simulink model "PMSM_z_domain_HDL"  (R2019b)
settings: Solver=ode1  StartTime=0.0  StopTime=2  FixedStep=1e-5  RelTol=1e-3
InitFcn:
  | %T=0.0000071
  | T = (1e-5)/2
  | 
  | flux=0.2068
values from neighbouring files (symbols this model uses):
  B = 0.0136    [Pmsm.m]
  J = 0.0027    [Pmsm.m]
  Kiq = double(Kiq)    [Pmsm.m]
  Kiw = double(Kiw)    [Pmsm.m]
  Kpq = double(Kpq)    [Pmsm.m]
  Kpw = double(Kpw)    [Pmsm.m]
  Lambda_m = 0.2026    [Pmsm.m]
  Ld = 19.75e-3    (= 0.01975)    [Pmsm.m]
  Lq = 22.5e-3    (= 0.0225)    [Pmsm.m]
  Ls = (Ld+Lq)/2    (= 0.021125)    [Pmsm.m]
  P = 8    [Pmsm.m]
  Rs = 1.477    [Pmsm.m]
  Vdc = 220    [Pmsm.m]
libraries: powerlib_meascontrol x3
settings Model: Creator=samfi  LastModifiedBy=samfi

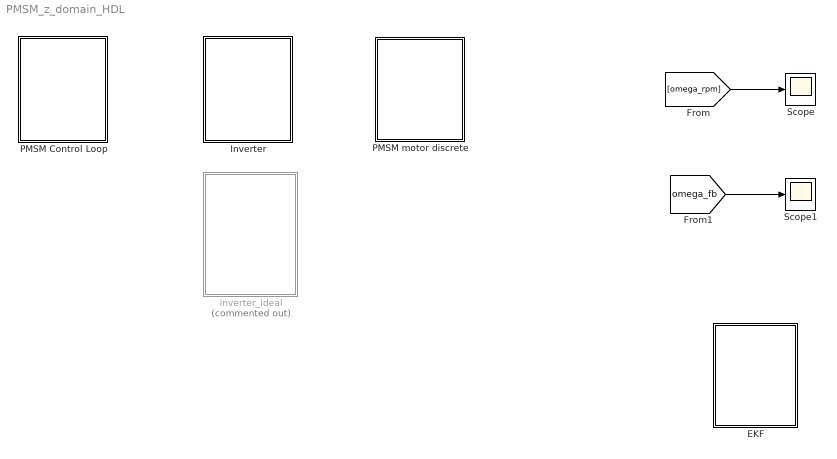
== system PMSM_z_domain_HDL ==
  EKF : Subsystem
  Inverter : Subsystem
  PMSM Control Loop : Subsystem
  PMSM motor discrete : Subsystem
  Scope : Scope
  Scope1 : Scope
  inverter_ideal : Subsystem  Commented=on
  wires:
  [omega_rpm] -> Scope/1
  [omega_fb] -> Scope1/1

== system PMSM_z_domain_HDL/EKF ==
  EKF good : Subsystem  Commented=on
  EKF good1 : Subsystem

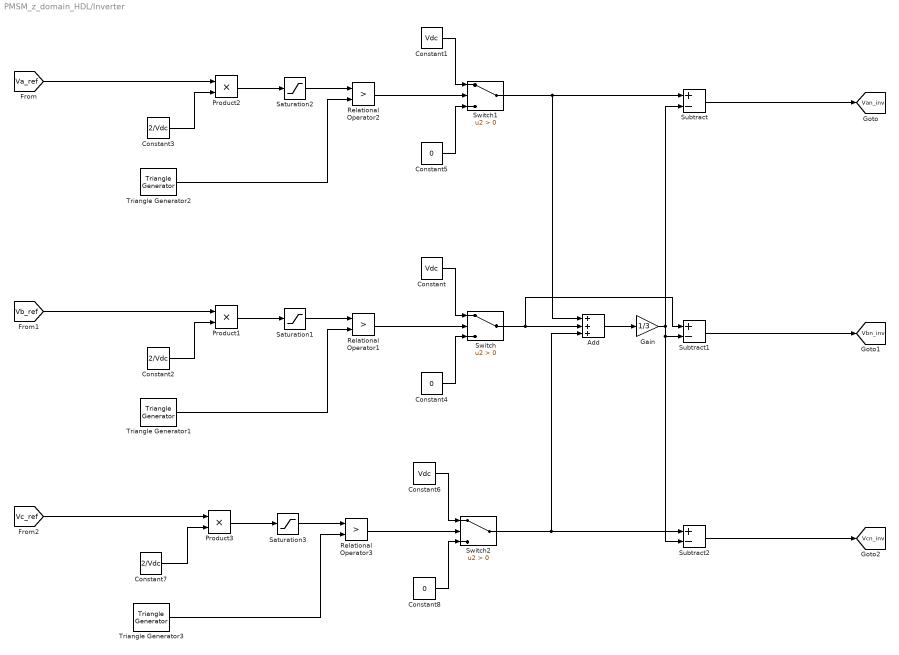
== system PMSM_z_domain_HDL/Inverter ==
  Add : Sum  Inputs=+++
  Constant : Constant  Value=Vdc
  Constant1 : Constant  Value=Vdc
  Constant2 : Constant  Value=2/Vdc
  Constant3 : Constant  Value=2/Vdc
  Constant4 : Constant  Value=0
  Constant5 : Constant  Value=0
  Constant6 : Constant  Value=Vdc
  Constant7 : Constant  Value=2/Vdc
  Constant8 : Constant  Value=0
  Gain : Gain  Gain=1/3
  Product1 : Product
  Product2 : Product
  Product3 : Product
  Relational Operator1 : RelationalOperator  Operator=>  OutDataTypeStr=boolean  RndMeth=Simplest
  Relational Operator2 : RelationalOperator  Operator=>  OutDataTypeStr=boolean  RndMeth=Simplest
  Relational Operator3 : RelationalOperator  Operator=>  OutDataTypeStr=boolean  RndMeth=Simplest
  Saturation1 : Saturate  UpperLimit=0.9  LowerLimit=-0.9
  Saturation2 : Saturate  UpperLimit=0.9  LowerLimit=-0.9
  Saturation3 : Saturate  UpperLimit=0.9  LowerLimit=-0.9
  Subtract : Sum  Inputs=+-
  Subtract1 : Sum  Inputs=+-
  Subtract2 : Sum  Inputs=+-
  Switch : Switch  Criteria=u2 > Threshold
  Switch1 : Switch  Criteria=u2 > Threshold
  Switch2 : Switch  Criteria=u2 > Threshold
  Triangle Generator1 : powerlib_meascontrol/Pulse & Signal Generators/Triangle Generator  Freq=1e4  Phase=0  Ts=0
      settings: SourceProductName=Simscape Electrical
  Triangle Generator2 : powerlib_meascontrol/Pulse & Signal Generators/Triangle Generator  Freq=1e4  Phase=0  Ts=0
      settings: SourceProductName=Simscape Electrical
  Triangle Generator3 : powerlib_meascontrol/Pulse & Signal Generators/Triangle Generator  Freq=1e4  Phase=0  Ts=0
      settings: SourceProductName=Simscape Electrical
  tag scope: Van_inv=global, Vbn_inv=global, Vcn_inv=global
  wires:
  Constant2/1 -> Product1/2
  Relational Operator1/1 -> Switch/2
  Constant5/1 -> Switch1/3
  Product1/1 -> Saturation1/1
  Constant1/1 -> Switch1/1
  Triangle Generator2/1 -> Relational Operator2/2
  [Va_ref] -> Product2/1
  Constant/1 -> Switch/1
  Relational Operator3/1 -> Switch2/2
  Triangle Generator1/1 -> Relational Operator1/2
  [Vb_ref] -> Product1/1
  Constant4/1 -> Switch/3
  [Vc_ref] -> Product3/1
  Constant3/1 -> Product2/2
  Triangle Generator3/1 -> Relational Operator3/2
  Product2/1 -> Saturation2/1
  Constant6/1 -> Switch2/1
  Constant8/1 -> Switch2/3
  Saturation2/1 -> Relational Operator2/1
  Product3/1 -> Saturation3/1
  Saturation3/1 -> Relational Operator3/1
  Constant7/1 -> Product3/2
  Relational Operator2/1 -> Switch1/2
  Saturation1/1 -> Relational Operator1/1
  Switch1/1 -> Subtract/1, Add/1
  Switch/1 -> Subtract1/1, Add/2
  Switch2/1 -> Subtract2/1, Add/3
  Subtract/1 -> [Van_inv]
  Add/1 -> Gain/1
  Gain/1 -> Subtract2/2, Subtract1/2, Subtract/2
  Subtract1/1 -> [Vbn_inv]
  Subtract2/1 -> [Vcn_inv]

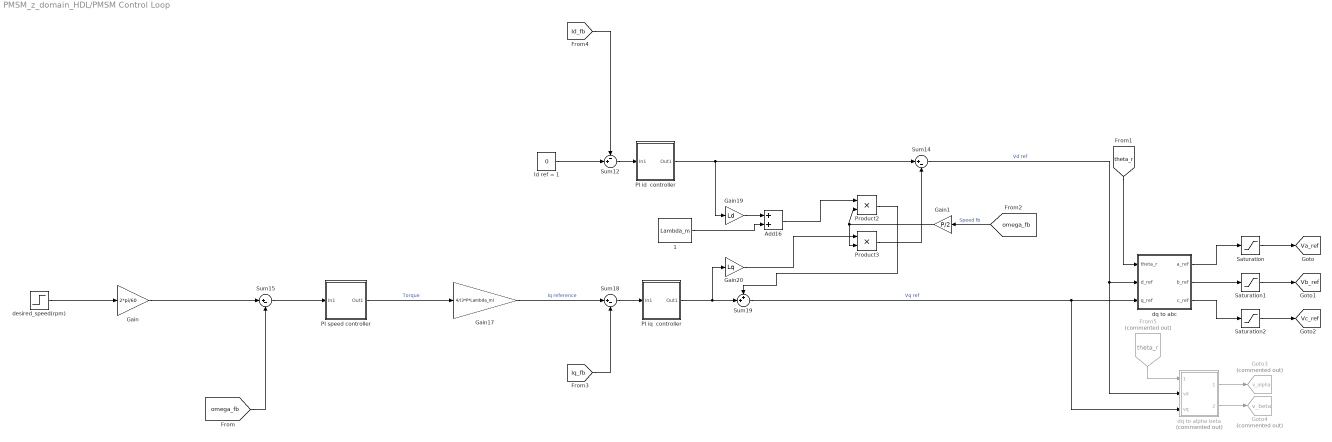
== system PMSM_z_domain_HDL/PMSM Control Loop ==
  " 1" : Constant  Value=Lambda_m
  Add16 : Sum
  From5 : From  Commented=on  GotoTag=theta_r  TagVisibility=global
  Gain : Gain  Gain=2*pi/60
  Gain1 : Gain  Gain=P/2
  Gain17 : Gain  Gain=4/(3*P*Lambda_m)
  Gain19 : Gain  Gain=Ld
  Gain20 : Gain  Gain=Lq
  Goto3 : Goto  Commented=on  GotoTag=v_alpha  TagVisibility=global
  Goto4 : Goto  Commented=on  GotoTag=v_beta  TagVisibility=global
  Id ref = 1 : Constant  Value=0
  PI id  controller : Subsystem
  PI iq  controller : Subsystem
  PI speed controller : Subsystem
  Product2 : Product
  Product3 : Product
  Saturation : Saturate  UpperLimit=200  LowerLimit=-200
  Saturation1 : Saturate  UpperLimit=200  LowerLimit=-200
  Saturation2 : Saturate  UpperLimit=200  LowerLimit=-200
  Sum12 : Sum  Inputs=-+|
  Sum14 : Sum  Inputs=|+-
  Sum15 : Sum  Inputs=|+-
  Sum18 : Sum  Inputs=|+-
  Sum19 : Sum  Inputs=++|
  desired_speed(rpm) : Step  Time=0.25  After=400  SampleTime=1e-4
  dq to abc : Subsystem
  dq to alpha beta : Subsystem  Commented=on
  tag scope: Va_ref=global, Vb_ref=global, Vc_ref=global
  wires:
  Product2/1 -> Sum19/1
  Add16/1 -> Product2/1
  Gain20/1 -> Product3/1
  Product3/1 -> Sum14/2
  Id ref = 1/1 -> Sum12/2
  PI iq  controller/1(Out1) -> Gain20/1, Sum19/2
  PI id  controller/1(Out1) -> Gain19/1, Sum14/1
  Sum14/1 -> dq to alpha beta/2(vd), dq to abc/2(d_ref)  "Vd ref"
  Gain19/1 -> Add16/1
  Sum18/1 -> PI iq  controller/1(In1)
  " 1"/1 -> Add16/2
  Gain17/1 -> Sum18/1  "Iq reference"
  Sum19/1 -> dq to alpha beta/3(vq), dq to abc/3(q_ref)  "Vq ref"
  [omega_fb] -> Sum15/2
  [theta_r] -> dq to abc/1(theta_r)
  [Iq_fb] -> Sum18/2
  [Id_fb] -> Sum12/1
  Saturation/1 -> [Va_ref]
  Saturation1/1 -> [Vb_ref]
  Saturation2/1 -> [Vc_ref]
  dq to abc/3(c_ref) -> Saturation2/1
  dq to abc/1(a_ref) -> Saturation/1
  dq to abc/2(b_ref) -> Saturation1/1
  Gain/1 -> Sum15/1
  [omega_fb] -> Gain1/1  "Speed fb"
  Gain1/1 -> Product3/2, Product2/2
  Sum12/1 -> PI id  controller/1(In1)
  Sum15/1 -> PI speed controller/1(In1)
  PI speed controller/1(Out1) -> Gain17/1  "Torque"
  dq to alpha beta/1(valpha) -> Goto3/1
  dq to alpha beta/2(vbeta) -> Goto4/1
  From5/1 -> dq to alpha beta/1(theta_r)
  desired_speed(rpm)/1 -> Gain/1

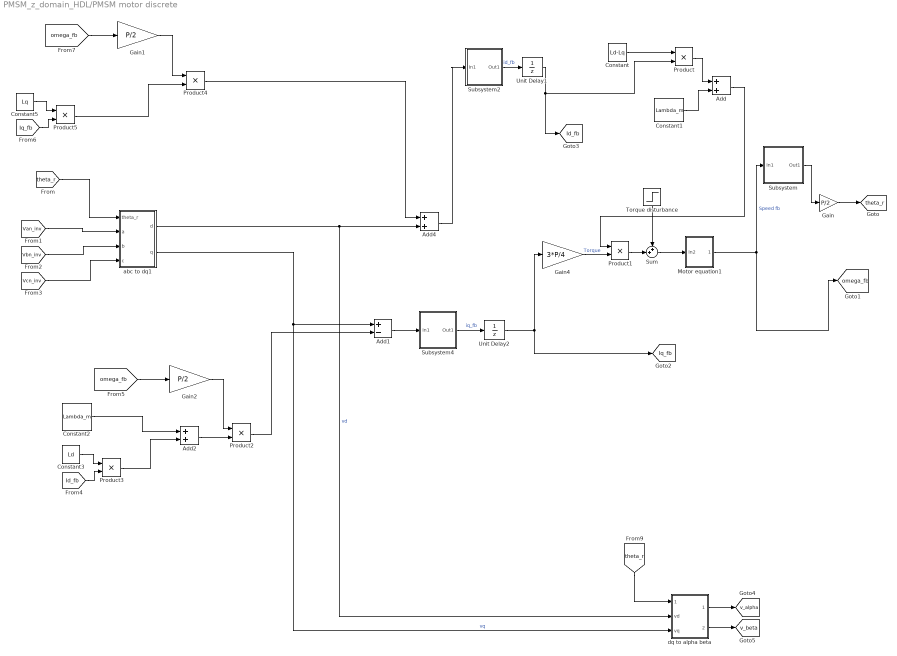
== system PMSM_z_domain_HDL/PMSM motor discrete ==
  Add : Sum
  Add1 : Sum  Inputs=+-
  Add2 : Sum
  Add4 : Sum
  Constant : Constant  Value=Ld-Lq
  Constant1 : Constant  Value=Lambda_m
  Constant2 : Constant  Value=Lambda_m
  Constant3 : Constant  Value=Ld
  Constant5 : Constant  Value=Lq
  Gain : Gain  Gain=P/2
  Gain1 : Gain  Gain=P/2
  Gain2 : Gain  Gain=P/2
  Gain4 : Gain  Gain=3*P/4
  Motor equation1 : Subsystem
  Product{,1..5} (6 alike) : Product
  Subsystem : Subsystem
  Subsystem2 : Subsystem
  Subsystem4 : Subsystem
  Sum : Sum  Inputs=++|
  Torque disturbance : Step  Time=2.5  After=0  SampleTime=0
  Unit Delay1 : UnitDelay  SampleTime=-1  HasFrameUpgradeWarning=on
  Unit Delay2 : UnitDelay  SampleTime=-1  HasFrameUpgradeWarning=on
  abc to dq1 : Subsystem
  dq to alpha beta : Subsystem
  tag scope: Id_fb=global, Iq_fb=global, omega_fb=global, theta_r=global, v_alpha=global, v_beta=global
  wires:
  Subsystem4/1(Out1) -> Unit Delay2/1  "iq_fb"
  [Vbn_inv] -> abc to dq1/3(b)
  Motor equation1/1(Out1) -> [omega_fb], Subsystem/1(In1)  "Speed fb"
  [Van_inv] -> abc to dq1/2(a)
  [Vcn_inv] -> abc to dq1/4(c)
  Subsystem2/1(Out1) -> Unit Delay1/1  "id_fb"
  Torque disturbance/1 -> Sum/1
  Sum/1 -> Motor equation1/1(In2)
  Constant/1 -> Product/1
  Product/1 -> Add/1
  Constant1/1 -> Add/2
  Gain4/1 -> Product1/2  "Torque"
  Product1/1 -> Sum/2
  Add/1 -> Product1/1
  Subsystem/1(Out1) -> Gain/1
  Gain/1 -> [theta_r]
  abc to dq1/2(q) -> dq to alpha beta/3(vq), Add1/1  "vq"
  Product2/1 -> Add1/2
  [omega_fb] -> Gain2/1
  Constant3/1 -> Product3/1
  [Id_fb] -> Product3/2
  Product3/1 -> Add2/2
  Constant2/1 -> Add2/1
  Add2/1 -> Product2/2
  [Iq_fb] -> Product5/2
  Product5/1 -> Product4/2
  Constant5/1 -> Product5/1
  abc to dq1/1(d) -> dq to alpha beta/2(vd), Add4/2  "vd"
  Product4/1 -> Add4/1
  [omega_fb] -> Gain1/1
  Gain1/1 -> Product4/1
  Gain2/1 -> Product2/1
  dq to alpha beta/1(valpha) -> [v_alpha]
  dq to alpha beta/2(vbeta) -> [v_beta]
  [theta_r] -> abc to dq1/1(theta_r)
  [theta_r] -> dq to alpha beta/1(theta_r)
  Add4/1 -> Subsystem2/1(In1)
  Add1/1 -> Subsystem4/1(In1)
  Unit Delay1/1 -> [Id_fb], Product/2
  Unit Delay2/1 -> Gain4/1, [Iq_fb]

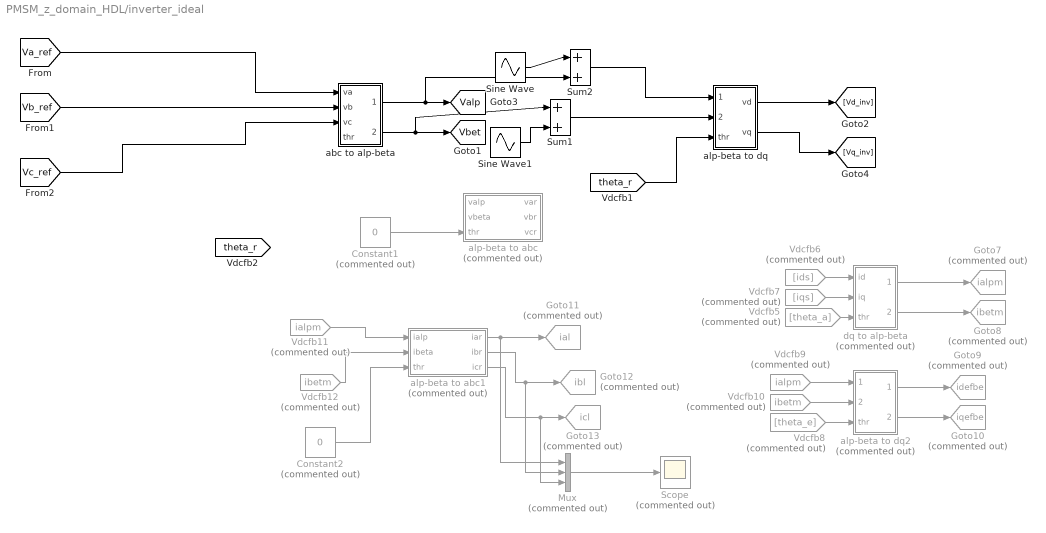
== system PMSM_z_domain_HDL/inverter_ideal ==
  Constant1 : Constant  Commented=on  Value=0
  Constant2 : Constant  Commented=on  Value=0
  Goto10 : Goto  Commented=on  GotoTag=iqefbe  TagVisibility=global
  Goto11 : Goto  Commented=on  GotoTag=ial  TagVisibility=global
  Goto12 : Goto  Commented=on  GotoTag=ibl  TagVisibility=global
  Goto13 : Goto  Commented=on  GotoTag=icl  TagVisibility=global
  Goto7 : Goto  Commented=on  GotoTag=ialpm  TagVisibility=global
  Goto8 : Goto  Commented=on  GotoTag=ibetm  TagVisibility=global
  Goto9 : Goto  Commented=on  GotoTag=idefbe  TagVisibility=global
  Mux : Mux  Commented=on  Inputs=3
  Scope : Scope  Commented=on
  Sine Wave : Sin  Amplitude=0  Frequency=2*pi*1000  SampleTime=0
  Sine Wave1 : Sin  Amplitude=0  Frequency=2*pi*1000  Phase=pi/2  SampleTime=0
  Sum1 : Sum  Inputs=|++
  Sum2 : Sum  Inputs=|++
  Vdcfb10 : From  Commented=on  GotoTag=ibetm  TagVisibility=global
      settings: CloseFcn=tagdialog Close
  Vdcfb11 : From  Commented=on  GotoTag=ialpm  TagVisibility=global
      settings: CloseFcn=tagdialog Close
  Vdcfb12 : From  Commented=on  GotoTag=ibetm  TagVisibility=global
      settings: CloseFcn=tagdialog Close
  Vdcfb5 : From  Commented=on  GotoTag=theta_a  TagVisibility=global
      settings: CloseFcn=tagdialog Close
  Vdcfb6 : From  Commented=on  GotoTag=ids  TagVisibility=global
      settings: CloseFcn=tagdialog Close
  Vdcfb7 : From  Commented=on  GotoTag=iqs  TagVisibility=global
      settings: CloseFcn=tagdialog Close
  Vdcfb8 : From  Commented=on  GotoTag=theta_e  TagVisibility=global
      settings: CloseFcn=tagdialog Close
  Vdcfb9 : From  Commented=on  GotoTag=ialpm  TagVisibility=global
      settings: CloseFcn=tagdialog Close
  abc to alp-beta : Subsystem
  alp-beta to abc : Subsystem  Commented=on
  alp-beta to abc1 : Subsystem  Commented=on
  alp-beta to dq : Subsystem
  alp-beta to dq2 : Subsystem  Commented=on
  dq to alp-beta : Subsystem  Commented=on
  tag scope: Valp=global, Vbet=global
  wires:
  abc to alp-beta/2(vbeta) -> [Vbet], Sum1/1
  abc to alp-beta/1(valp) -> [Valp], Sum2/2
  ? -> abc to alp-beta/4(thr)
  [Vb_ref] -> abc to alp-beta/2(vb)
  [Va_ref] -> abc to alp-beta/1(va)
  [Vc_ref] -> abc to alp-beta/3(vc)
  [theta_r] -> alp-beta to dq/3(thr)
  Vdcfb5/1 -> dq to alp-beta/3(thr)
  alp-beta to dq/1(vd) -> [Vd_inv]
  alp-beta to dq/2(vq) -> [Vq_inv]
  Vdcfb6/1 -> dq to alp-beta/1(id)
  Vdcfb7/1 -> dq to alp-beta/2(iq)
  Vdcfb8/1 -> alp-beta to dq2/3(thr)
  dq to alp-beta/1(ialp) -> Goto7/1
  dq to alp-beta/2(ibet) -> Goto8/1
  Vdcfb9/1 -> alp-beta to dq2/1(ialp)
  Vdcfb10/1 -> alp-beta to dq2/2(ibet)
  alp-beta to dq2/1(ide) -> Goto9/1
  alp-beta to dq2/2(iqe) -> Goto10/1
  Sine Wave/1 -> Sum2/1
  Sum2/1 -> alp-beta to dq/1(valp)
  Sine Wave1/1 -> Sum1/2
  Sum1/1 -> alp-beta to dq/2(vbet)
  Vdcfb11/1 -> alp-beta to abc1/1(ialp)
  Vdcfb12/1 -> alp-beta to abc1/2(ibeta)
  Constant2/1 -> alp-beta to abc1/3(thr)
  alp-beta to abc1/1(iar) -> Goto11/1, Mux/1
  alp-beta to abc1/2(ibr) -> Goto12/1, Mux/2
  alp-beta to abc1/3(icr) -> Goto13/1, Mux/3
  Mux/1 -> Scope/1
  Constant1/1 -> alp-beta to abc/3(thr)

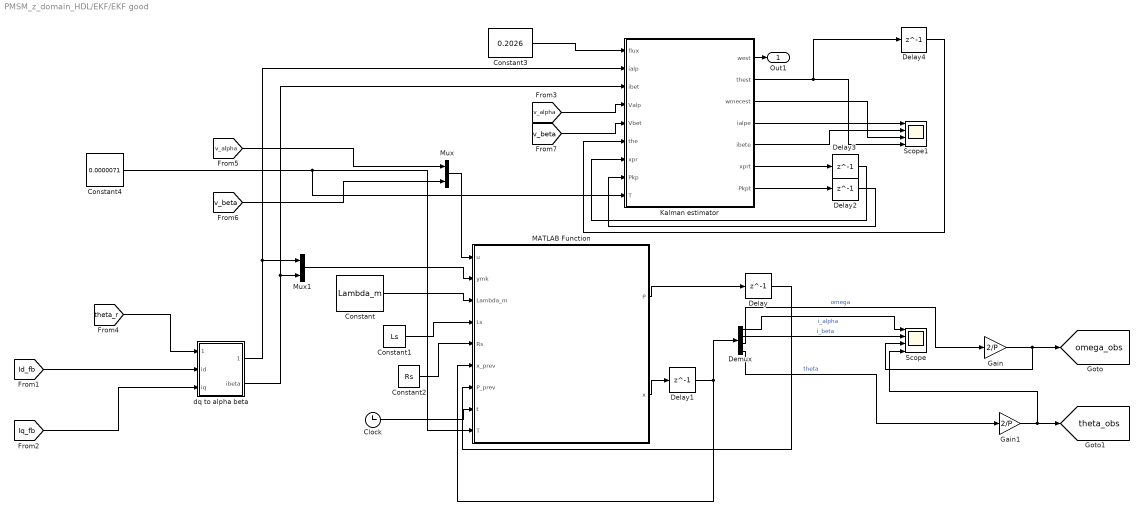
== system PMSM_z_domain_HDL/EKF/EKF good ==
  Clock : Clock
  Constant : Constant  Value=Lambda_m
  Constant1 : Constant  Value=Ls
  Constant2 : Constant  Value=Rs
  Constant3 : Constant  Value=0.2026
  Constant4 : Constant  Value=0.0000071
  Delay{,1..4} (5 alike) : Delay  DelayLength=1  InitialCondition=0
  Demux : Demux
  Gain : Gain  Gain=2/P
  Gain1 : Gain  Gain=2/P
  Kalman estimator : Subsystem  SystemSampleTime=1e-4
  MATLAB Function : MATLAB Function  TreatAsAtomicUnit=on
  Mux : Mux  Inputs=2
  Mux1 : Mux  Inputs=2
  Scope : Scope  NumInputPorts=4
  Scope1 : Scope  NumInputPorts=4
  dq to alpha beta : Subsystem
  Out1 : Outport
  tag scope: omega_obs=global, theta_obs=global
  wires:
  Kalman estimator/3(wmecest) -> Scope1/3
  dq to alpha beta/2(ibeta) -> Kalman estimator/3(ibet), Mux1/2
  Delay/1 -> MATLAB Function/7(P_prev)
  Constant/1 -> MATLAB Function/3(Lambda_m)
  [v_beta] -> Kalman estimator/5(Vbet)
  Delay2/1 -> Kalman estimator/8(Pkp)
  Kalman estimator/2(thest) -> Delay4/1, Scope1/4
  Mux/1 -> MATLAB Function/1(u)
  [v_alpha] -> Kalman estimator/4(Valp)
  Demux/3 -> Gain/1  "omega"
  Kalman estimator/6(xprt) -> Delay3/1
  Delay3/1 -> Kalman estimator/7(xpr)
  Gain1/1 -> Scope/4, [theta_obs]
  dq to alpha beta/1(ialpha) -> Kalman estimator/2(ialp), Mux1/1
  Kalman estimator/4(ialpe) -> Scope1/1
  Kalman estimator/7(Pkpt) -> Delay2/1
  Mux1/1 -> MATLAB Function/2(ymk)
  Kalman estimator/1(west) -> Out1/1
  Kalman estimator/5(ibete) -> Scope1/2
  Delay4/1 -> Kalman estimator/6(the)
  Gain/1 -> Scope/3, [omega_obs]
  Constant2/1 -> MATLAB Function/5(Rs)
  Clock/1 -> MATLAB Function/8(t)
  Constant3/1 -> Kalman estimator/1(flux)
  [Id_fb] -> dq to alpha beta/2(id)
  MATLAB Function/2(x) -> Delay1/1
  [v_beta] -> Mux/2
  [v_alpha] -> Mux/1
  Constant4/1 -> MATLAB Function/9(T), Kalman estimator/9(T)
  Delay1/1 -> Demux/1, MATLAB Function/6(x_prev)
  Demux/4 -> Gain1/1  "theta"
  Demux/2 -> Scope/2  "i_beta"
  [Iq_fb] -> dq to alpha beta/3(iq)
  Demux/1 -> Scope/1  "i_alpha"
  MATLAB Function/1(P) -> Delay/1
  Constant1/1 -> MATLAB Function/4(Ls)
  [theta_r] -> dq to alpha beta/1(theta_r)

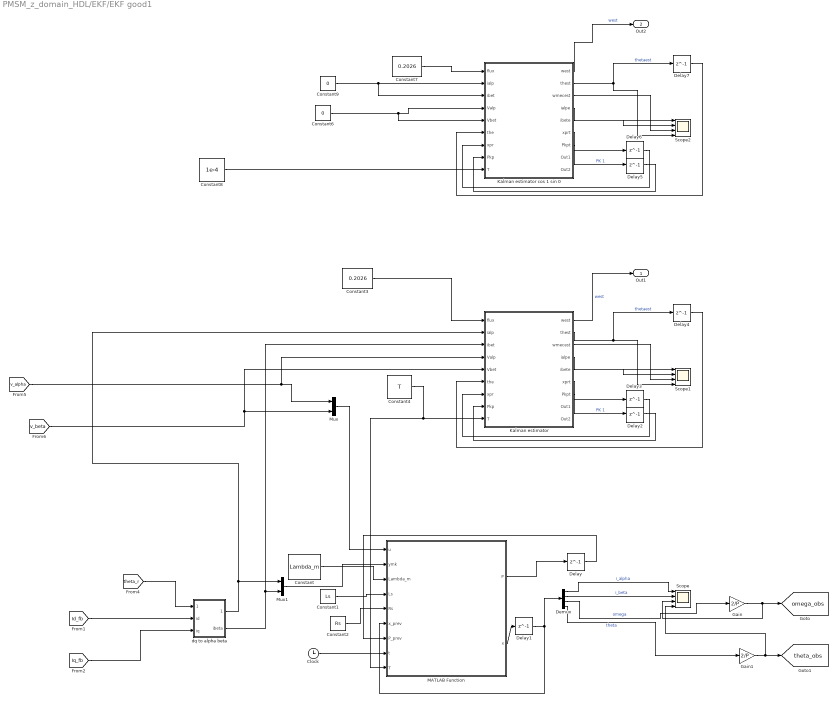
== system PMSM_z_domain_HDL/EKF/EKF good1 ==
  Clock : Clock
  Constant : Constant  Value=Lambda_m
  Constant1 : Constant  Value=Ls
  Constant2 : Constant  Value=Rs
  Constant3 : Constant  Value=0.2026
  Constant4 : Constant  Value=T  SampleTime=1e-4
  Constant6 : Constant  Value=0  SampleTime=10e-5
  Constant7 : Constant  Value=0.2026
  Constant8 : Constant  Value=1e-4
  Constant9 : Constant  Value=0  SampleTime=10e-5
  Delay{,1..7} (8 alike) : Delay  DelayLength=1  InitialCondition=0
  Demux : Demux
  Gain : Gain  Gain=2/P
  Gain1 : Gain  Gain=2/P
  Kalman estimator : Subsystem  SystemSampleTime=1e-4
  Kalman estimator cos 1 sin 0 : Subsystem  SystemSampleTime=1e-4
  MATLAB Function : MATLAB Function  TreatAsAtomicUnit=on
  Mux : Mux  Inputs=2
  Mux1 : Mux  Inputs=2
  Scope : Scope  NumInputPorts=4
  Scope1 : Scope  NumInputPorts=4
  Scope2 : Scope  NumInputPorts=4
  dq to alpha beta : Subsystem
  Out1 : Outport
  Out2 : Outport  Port=2
  tag scope: omega_obs=global, theta_obs=global
  wires:
  [theta_r] -> dq to alpha beta/1(theta_r)
  Constant1/1 -> MATLAB Function/4(Ls)
  MATLAB Function/1(P) -> Delay/1
  Demux/1 -> Scope/1  "i_alpha"
  [Iq_fb] -> dq to alpha beta/3(iq)
  Demux/2 -> Scope/2  "i_beta"
  Demux/4 -> Gain1/1  "theta"
  Delay1/1 -> MATLAB Function/6(x_prev), Demux/1
  Constant4/1 -> MATLAB Function/9(T), Kalman estimator/9(T)
  [v_alpha] -> Mux/1, Kalman estimator/4(Valp)
  [v_beta] -> Kalman estimator/5(Vbet), Mux/2
  MATLAB Function/2(x) -> Delay1/1
  [Id_fb] -> dq to alpha beta/2(id)
  Constant3/1 -> Kalman estimator/1(flux)
  Clock/1 -> MATLAB Function/8(t)
  Constant2/1 -> MATLAB Function/5(Rs)
  Gain/1 -> [omega_obs], Scope/3
  Delay4/1 -> Kalman estimator/6(the)
  Kalman estimator/5(ibete) -> Scope1/2
  Kalman estimator/1(west) -> Out1/1  "west"
  Mux1/1 -> MATLAB Function/2(ymk)
  Kalman estimator/7(Pkpt) -> Delay2/1  "PK 1"
  Kalman estimator/4(ialpe) -> Scope1/1
  dq to alpha beta/1(ialpha) -> Kalman estimator/2(ialp), Mux1/1
  Gain1/1 -> [theta_obs], Scope/4
  Delay3/1 -> Kalman estimator/7(xpr)
  Kalman estimator/6(xprt) -> Delay3/1
  Demux/3 -> Gain/1  "omega"
  Mux/1 -> MATLAB Function/1(u)
  Kalman estimator/2(thest) -> Scope1/4, Delay4/1  "thetaest"
  Delay2/1 -> Kalman estimator/8(Pkp)
  Constant/1 -> MATLAB Function/3(Lambda_m)
  Delay/1 -> MATLAB Function/7(P_prev)
  dq to alpha beta/2(ibeta) -> Kalman estimator/3(ibet), Mux1/2
  Kalman estimator/3(wmecest) -> Scope1/3
  Constant6/1 -> Kalman estimator cos 1 sin 0/4(Valp), Kalman estimator cos 1 sin 0/5(Vbet)
  Constant9/1 -> Kalman estimator cos 1 sin 0/3(ibet), Kalman estimator cos 1 sin 0/2(ialp)
  Kalman estimator cos 1 sin 0/3(wmecest) -> Scope2/3
  Delay5/1 -> Kalman estimator cos 1 sin 0/8(Pkp)
  Kalman estimator cos 1 sin 0/2(thest) -> Scope2/4, Delay7/1  "thetaest"
  Kalman estimator cos 1 sin 0/6(xprt) -> Delay6/1
  Delay6/1 -> Kalman estimator cos 1 sin 0/7(xpr)
  Kalman estimator cos 1 sin 0/4(ialpe) -> Scope2/1
  Kalman estimator cos 1 sin 0/7(Pkpt) -> Delay5/1  "PK 1"
  Kalman estimator cos 1 sin 0/1(west) -> Out2/1  "west"
  Kalman estimator cos 1 sin 0/5(ibete) -> Scope2/2
  Delay7/1 -> Kalman estimator cos 1 sin 0/6(the)
  Constant7/1 -> Kalman estimator cos 1 sin 0/1(flux)
  Constant8/1 -> Kalman estimator cos 1 sin 0/9(T)

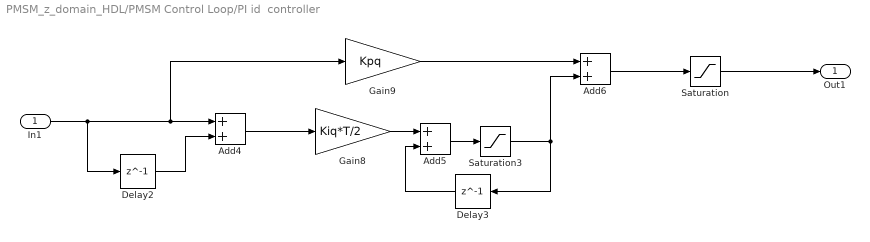
== system PMSM_z_domain_HDL/PMSM Control Loop/PI id  controller ==
  In1 : Inport
  Add4 : Sum
  Add5 : Sum
  Add6 : Sum
  Delay2 : Delay  DelayLength=1
  Delay3 : Delay  DelayLength=1
  Gain8 : Gain  Gain=Kiq*T/2
  Gain9 : Gain  Gain=Kpq
  Saturation : Saturate  UpperLimit=220  LowerLimit=-220
  Saturation3 : Saturate  UpperLimit=200  LowerLimit=-200
  Out1 : Outport
  wires:
  Gain8/1 -> Add5/1
  Delay2/1 -> Add4/2
  Add5/1 -> Saturation3/1
  Add4/1 -> Gain8/1
  Saturation3/1 -> Delay3/1, Add6/2
  In1/1 -> Add4/1, Gain9/1, Delay2/1
  Gain9/1 -> Add6/1
  Delay3/1 -> Add5/2
  Add6/1 -> Saturation/1
  Saturation/1 -> Out1/1

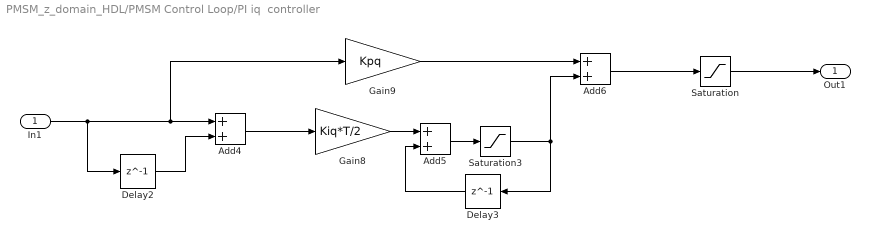
== system PMSM_z_domain_HDL/PMSM Control Loop/PI iq  controller ==
  In1 : Inport
  Add4 : Sum
  Add5 : Sum
  Add6 : Sum
  Delay2 : Delay  DelayLength=1
  Delay3 : Delay  DelayLength=1
  Gain8 : Gain  Gain=Kiq*T/2
  Gain9 : Gain  Gain=Kpq
  Saturation : Saturate  UpperLimit=220  LowerLimit=-220
  Saturation3 : Saturate  UpperLimit=200  LowerLimit=-200
  Out1 : Outport
  wires:
  Delay3/1 -> Add5/2
  Gain9/1 -> Add6/1
  In1/1 -> Delay2/1, Gain9/1, Add4/1
  Saturation3/1 -> Add6/2, Delay3/1
  Add4/1 -> Gain8/1
  Add5/1 -> Saturation3/1
  Delay2/1 -> Add4/2
  Gain8/1 -> Add5/1
  Add6/1 -> Saturation/1
  Saturation/1 -> Out1/1

== system PMSM_z_domain_HDL/PMSM Control Loop/PI speed controller ==
  In1 : Inport
  Add4 : Sum
  Add5 : Sum
  Add6 : Sum
  Delay2 : Delay  DelayLength=1
  Delay3 : Delay  DelayLength=1
  Gain8 : Gain  Gain=Kiw*T/2
  Gain9 : Gain  Gain=Kpw
  Saturation : Saturate  UpperLimit=10  LowerLimit=-10
  Saturation1 : Saturate  UpperLimit=10  LowerLimit=-10
  Out1 : Outport
  wires:
  Gain9/1 -> Add6/1
  Delay2/1 -> Add4/2
  Gain8/1 -> Add5/1
  Add5/1 -> Saturation/1
  In1/1 -> Delay2/1, Gain9/1, Add4/1
  Saturation/1 -> Add6/2, Delay3/1
  Add4/1 -> Gain8/1
  Delay3/1 -> Add5/2
  Add6/1 -> Saturation1/1
  Saturation1/1 -> Out1/1

== system PMSM_z_domain_HDL/PMSM Control Loop/dq to abc ==
  theta_r : Inport
  d_ref : Inport  Port=2
  q_ref : Inport  Port=3
  Mux : Mux  Inputs=3
  a : Fcn  Expr=cos(u(1))*u(2)-sin(u(1))*u(3)
  b : Fcn  Expr=cos(u(1)-2*pi/3)*u(2)-sin(u(1)-2*pi/3)*u(3)
  c : Fcn  Expr=cos(u(1)+2*pi/3)*u(2)-sin(u(1)+2*pi/3)*u(3)
  a_ref : Outport
  b_ref : Outport  Port=2
  c_ref : Outport  Port=3
  wires:
  d_ref/1 -> Mux/2
  Mux/1 -> c/1, b/1, a/1
  c/1 -> c_ref/1
  theta_r/1 -> Mux/1
  b/1 -> b_ref/1
  a/1 -> a_ref/1
  q_ref/1 -> Mux/3

== system PMSM_z_domain_HDL/PMSM Control Loop/dq to alpha beta ==
  theta_r : Inport
  vd : Inport  Port=2
  vq : Inport  Port=3
  Fcn : Fcn  Expr=cos(u(1))*u(2)-sin(u(1))*u(3)
  Fcn1 : Fcn  Expr=sin(u(1))*u(2)+cos(u(1))*u(3)
  Mux : Mux  Inputs=3
  valpha : Outport
  vbeta : Outport  Port=2
  wires:
  Mux/1 -> Fcn/1, Fcn1/1
  vq/1 -> Mux/3
  theta_r/1 -> Mux/1
  Fcn1/1 -> vbeta/1
  vd/1 -> Mux/2
  Fcn/1 -> valpha/1

== system PMSM_z_domain_HDL/PMSM motor discrete/Motor equation1 ==
  In2 : Inport
  Add7 : Sum
  Add8 : Sum  Inputs=+-
  Delay2 : Delay  DelayLength=1
  Delay4 : Delay  DelayLength=1
  Gain1 : Gain  Gain=1/(B+(2*J/T))
  Gain2 : Gain  Gain=B-(2*J/T)
  Out1 : Outport
  wires:
  Add7/1 -> Add8/1
  Gain1/1 -> Out1/1, Delay2/1
  Delay2/1 -> Gain2/1
  Add8/1 -> Gain1/1
  Gain2/1 -> Add8/2
  In2/1 -> Delay4/1, Add7/1
  Delay4/1 -> Add7/2

== system PMSM_z_domain_HDL/PMSM motor discrete/Subsystem ==
  In1 : Inport
  Add1 : Sum
  Add2 : Sum
  Delay1 : Delay  DelayLength=1
  Delay4 : Delay  DelayLength=1
  Gain : Gain  Gain=T/2
  Out1 : Outport
  wires:
  In1/1 -> Delay4/1, Add1/1
  Delay1/1 -> Add2/2
  Add2/1 -> Out1/1, Delay1/1
  Delay4/1 -> Add1/2
  Add1/1 -> Gain/1
  Gain/1 -> Add2/1

== system PMSM_z_domain_HDL/PMSM motor discrete/Subsystem2 ==
  In1 : Inport
  Add7 : Sum
  Add8 : Sum  Inputs=+-
  Delay2 : Delay  DelayLength=1
  Delay4 : Delay  DelayLength=1
  Gain1 : Gain  Gain=1/(Rs+(2*Ld/T))
  Gain2 : Gain  Gain=Rs-(2*Ld/T)
  Out1 : Outport
  wires:
  Add8/1 -> Gain1/1
  In1/1 -> Add7/1, Delay4/1
  Gain2/1 -> Add8/2
  Delay2/1 -> Gain2/1
  Delay4/1 -> Add7/2
  Add7/1 -> Add8/1
  Gain1/1 -> Out1/1, Delay2/1

== system PMSM_z_domain_HDL/PMSM motor discrete/Subsystem4 ==
  In1 : Inport
  Add7 : Sum
  Add8 : Sum  Inputs=+-
  Delay2 : Delay  DelayLength=1
  Delay4 : Delay  DelayLength=1
  Gain1 : Gain  Gain=1/(Rs+(2*Lq/T))
  Gain2 : Gain  Gain=Rs-(2*Lq/T)
  Out1 : Outport
  wires:
  Add8/1 -> Gain1/1
  Gain1/1 -> Delay2/1, Out1/1
  Add7/1 -> Add8/1
  Delay4/1 -> Add7/2
  Delay2/1 -> Gain2/1
  Gain2/1 -> Add8/2
  In1/1 -> Delay4/1, Add7/1

== system PMSM_z_domain_HDL/PMSM motor discrete/abc to dq1 ==
  theta_r : Inport
  a : Inport  Port=2
  b : Inport  Port=3
  c : Inport  Port=4
  Fcn : Fcn  Expr=(2/3)*(cos(u(1))*u(2)+cos(u(1)-2*pi/3)*u(3)+cos(u(1)+2*pi/3)*u(4))
  Fcn1 : Fcn  Expr=(2/3)*(-sin(u(1))*u(2)-sin(u(1)-2*pi/3)*u(3)-sin(u(1)+2*pi/3)*u(4))
  Mux : Mux
  d : Outport
  q : Outport  Port=2
  wires:
  a/1 -> Mux/2
  c/1 -> Mux/4
  theta_r/1 -> Mux/1
  Mux/1 -> Fcn/1, Fcn1/1
  b/1 -> Mux/3
  Fcn/1 -> d/1
  Fcn1/1 -> q/1

== system PMSM_z_domain_HDL/PMSM motor discrete/dq to alpha beta ==
  theta_r : Inport
  vd : Inport  Port=2
  vq : Inport  Port=3
  Fcn : Fcn  Expr=cos(u(1))*u(2)-sin(u(1))*u(3)
  Fcn1 : Fcn  Expr=sin(u(1))*u(2)+cos(u(1))*u(3)
  Mux : Mux  Inputs=3
  valpha : Outport
  vbeta : Outport  Port=2
  wires:
  Mux/1 -> Fcn/1, Fcn1/1
  vq/1 -> Mux/3
  theta_r/1 -> Mux/1
  Fcn1/1 -> vbeta/1
  vd/1 -> Mux/2
  Fcn/1 -> valpha/1

== system PMSM_z_domain_HDL/inverter_ideal/abc to alp-beta ==
  va : Inport
  vb : Inport  Port=2
  vc : Inport  Port=3
  thr : Inport  Port=4
  Fcn : Fcn  Expr=((u(1)*cos(u(4)))+(u(2)*cos(u(4)-2*pi/3))+(u(3)*cos(u(4)+(2*pi/3))))*(2/3)
  Fcn1 : Fcn  Expr=-((u(1)*sin(u(4)))+(u(2)*sin(u(4)-(2*pi/3)))+(u(3)*sin(u(4)+(2*pi/3))))*(2/3)
  Mux : Mux
  Unit Delay1 : UnitDelay  SampleTime=-1
  Unit Delay3 : UnitDelay  SampleTime=-1
  valp : Outport
  vbeta : Outport  Port=2
  wires:
  Fcn1/1 -> Unit Delay1/1
  Fcn/1 -> Unit Delay3/1
  Mux/1 -> Fcn1/1, Fcn/1
  va/1 -> Mux/1
  thr/1 -> Mux/4
  vc/1 -> Mux/3
  vb/1 -> Mux/2
  Unit Delay3/1 -> valp/1
  Unit Delay1/1 -> vbeta/1

== system PMSM_z_domain_HDL/inverter_ideal/alp-beta to abc ==
  valp : Inport
  vbeta : Inport  Port=2
  thr : Inport  Port=3
  Fcn : Fcn  Expr=u(1)*cos(u(3))-u(2)*sin(u(3))
  Fcn1 : Fcn  Expr=u(1)*cos(u(3)-2*pi/3)-u(2)*sin(u(3)-2*pi/3)
  Fcn2 : Fcn  Expr=u(1)*cos(u(3)+2*pi/3)-u(2)*sin(u(3)+2*pi/3)
  Mux : Mux  Inputs=3
  var : Outport
  vbr : Outport  Port=2
  vcr : Outport  Port=3
  wires:
  valp/1 -> Mux/1
  vbeta/1 -> Mux/2
  thr/1 -> Mux/3
  Mux/1 -> Fcn/1, Fcn1/1, Fcn2/1
  Fcn/1 -> var/1
  Fcn1/1 -> vbr/1
  Fcn2/1 -> vcr/1

== system PMSM_z_domain_HDL/inverter_ideal/alp-beta to abc1 ==
  ialp : Inport
  ibeta : Inport  Port=2
  thr : Inport  Port=3
  Fcn : Fcn  Expr=u(1)*cos(u(3))-u(2)*sin(u(3))
  Fcn1 : Fcn  Expr=u(1)*cos(u(3)-2*pi/3)-u(2)*sin(u(3)-2*pi/3)
  Fcn2 : Fcn  Expr=u(1)*cos(u(3)+2*pi/3)-u(2)*sin(u(3)+2*pi/3)
  Mux : Mux  Inputs=3
  iar : Outport
  ibr : Outport  Port=2
  icr : Outport  Port=3
  wires:
  Fcn2/1 -> icr/1
  Fcn1/1 -> ibr/1
  Fcn/1 -> iar/1
  Mux/1 -> Fcn2/1, Fcn1/1, Fcn/1
  thr/1 -> Mux/3
  ibeta/1 -> Mux/2
  ialp/1 -> Mux/1

== system PMSM_z_domain_HDL/inverter_ideal/alp-beta to dq ==
  valp : Inport
  vbet : Inport  Port=2
  thr : Inport  Port=3
  Fcn : Fcn  Expr=(u(1)*cos(u(3)))+(u(2)*sin(u(3)))
  Fcn1 : Fcn  Expr=-(u(1)*sin(u(3)))+(u(2)*cos(u(3)))
  Mux : Mux  Inputs=3
  vd : Outport
  vq : Outport  Port=2
  wires:
  vbet/1 -> Mux/2
  thr/1 -> Mux/3
  valp/1 -> Mux/1
  Mux/1 -> Fcn/1, Fcn1/1
  Fcn/1 -> vd/1
  Fcn1/1 -> vq/1

== system PMSM_z_domain_HDL/inverter_ideal/alp-beta to dq2 ==
  ialp : Inport
  ibet : Inport  Port=2
  thr : Inport  Port=3
  Fcn : Fcn  Expr=(u(1)*cos(u(3)))+(u(2)*sin(u(3)))
  Fcn1 : Fcn  Expr=-(u(1)*sin(u(3)))+(u(2)*cos(u(3)))
  Mux : Mux  Inputs=3
  ide : Outport
  iqe : Outport  Port=2
  wires:
  ibet/1 -> Mux/2
  thr/1 -> Mux/3
  ialp/1 -> Mux/1
  Mux/1 -> Fcn/1, Fcn1/1
  Fcn/1 -> ide/1
  Fcn1/1 -> iqe/1

== system PMSM_z_domain_HDL/inverter_ideal/dq to alp-beta ==
  id : Inport
  iq : Inport  Port=2
  thr : Inport  Port=3
  Fcn : Fcn  Expr=(u(1)*cos(u(3)))-(u(2)*sin(u(3)))
  Fcn1 : Fcn  Expr=(u(1)*sin(u(3)))+(u(2)*cos(u(3)))
  Mux : Mux  Inputs=3
  ialp : Outport
  ibet : Outport  Port=2
  wires:
  Fcn1/1 -> ibet/1
  Fcn/1 -> ialp/1
  Mux/1 -> Fcn1/1, Fcn/1
  id/1 -> Mux/1
  thr/1 -> Mux/3
  iq/1 -> Mux/2

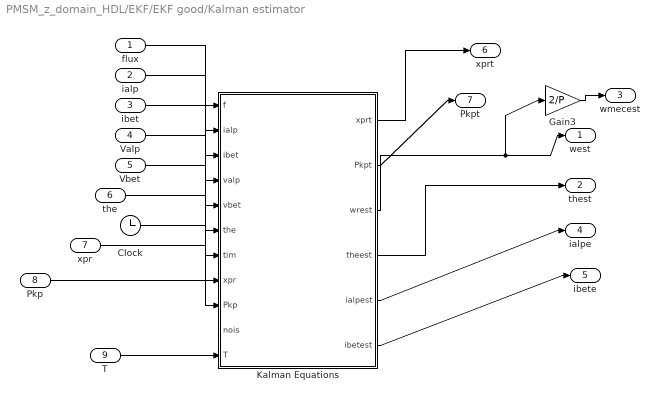
== system PMSM_z_domain_HDL/EKF/EKF good/Kalman estimator ==
  flux : Inport
  ialp : Inport  Port=2
  ibet : Inport  Port=3
  Valp : Inport  Port=4
  Vbet : Inport  Port=5
  the : Inport  Port=6
  xpr : Inport  Port=7
  Pkp : Inport  Port=8
  T : Inport  Port=9
  Clock : Clock
  Gain3 : Gain  Gain=2/P
  Kalman Equations : MATLAB Function  TreatAsAtomicUnit=on
  west : Outport
  thest : Outport  Port=2
  wmecest : Outport  Port=3
  ialpe : Outport  Port=4
  ibete : Outport  Port=5
  xprt : Outport  Port=6
  Pkpt : Outport  Port=7
  wires:
  flux/1 -> Kalman Equations/1(f)
  Valp/1 -> Kalman Equations/4(valp)
  Vbet/1 -> Kalman Equations/5(vbet)
  Clock/1 -> Kalman Equations/7(tim)
  Kalman Equations/3(wrest) -> west/1, Gain3/1
  Kalman Equations/4(theest) -> thest/1
  Gain3/1 -> wmecest/1
  ialp/1 -> Kalman Equations/2(ialp)
  ibet/1 -> Kalman Equations/3(ibet)
  Kalman Equations/5(ialpest) -> ialpe/1
  Kalman Equations/6(ibetest) -> ibete/1
  Kalman Equations/1(xprt) -> xprt/1
  Kalman Equations/2(Pkpt) -> Pkpt/1
  the/1 -> Kalman Equations/6(the)
  xpr/1 -> Kalman Equations/8(xpr)
  Pkp/1 -> Kalman Equations/9(Pkp)
  T/1 -> Kalman Equations/11(T)

== system PMSM_z_domain_HDL/EKF/EKF good/dq to alpha beta ==
  theta_r : Inport
  id : Inport  Port=2
  iq : Inport  Port=3
  Fcn : Fcn  Expr=cos(u(1))*u(2)-sin(u(1))*u(3)
  Fcn1 : Fcn  Expr=sin(u(1))*u(2)+cos(u(1))*u(3)
  Mux : Mux  Inputs=3
  ialpha : Outport
  ibeta : Outport  Port=2
  wires:
  Mux/1 -> Fcn/1, Fcn1/1
  iq/1 -> Mux/3
  theta_r/1 -> Mux/1
  Fcn1/1 -> ibeta/1
  id/1 -> Mux/2
  Fcn/1 -> ialpha/1

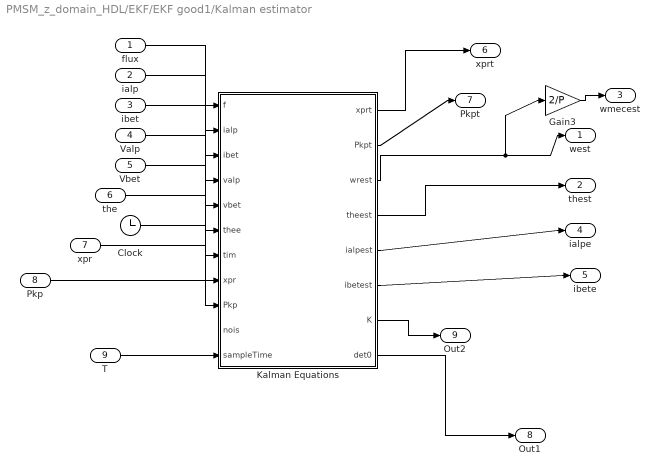
== system PMSM_z_domain_HDL/EKF/EKF good1/Kalman estimator ==
  flux : Inport
  ialp : Inport  Port=2
  ibet : Inport  Port=3
  Valp : Inport  Port=4
  Vbet : Inport  Port=5
  the : Inport  Port=6
  xpr : Inport  Port=7
  Pkp : Inport  Port=8
  T : Inport  Port=9
  Clock : Clock
  Gain3 : Gain  Gain=2/P
  Kalman Equations : MATLAB Function  TreatAsAtomicUnit=on
  west : Outport
  thest : Outport  Port=2
  wmecest : Outport  Port=3
  ialpe : Outport  Port=4
  ibete : Outport  Port=5
  xprt : Outport  Port=6
  Pkpt : Outport  Port=7
  Out1 : Outport  Port=8
  Out2 : Outport  Port=9
  wires:
  T/1 -> Kalman Equations/11(sampleTime)
  Pkp/1 -> Kalman Equations/9(Pkp)
  xpr/1 -> Kalman Equations/8(xpr)
  the/1 -> Kalman Equations/6(thee)
  Kalman Equations/2(Pkpt) -> Pkpt/1
  Kalman Equations/1(xprt) -> xprt/1
  Kalman Equations/6(ibetest) -> ibete/1
  Kalman Equations/5(ialpest) -> ialpe/1
  ibet/1 -> Kalman Equations/3(ibet)
  ialp/1 -> Kalman Equations/2(ialp)
  Gain3/1 -> wmecest/1
  Kalman Equations/4(theest) -> thest/1
  Kalman Equations/3(wrest) -> Gain3/1, west/1
  Clock/1 -> Kalman Equations/7(tim)
  Vbet/1 -> Kalman Equations/5(vbet)
  Valp/1 -> Kalman Equations/4(valp)
  flux/1 -> Kalman Equations/1(f)
  Kalman Equations/8(det0) -> Out1/1
  Kalman Equations/7(K) -> Out2/1

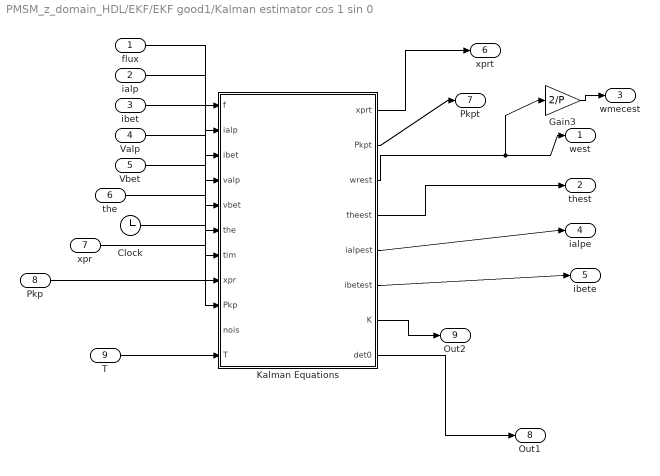
== system PMSM_z_domain_HDL/EKF/EKF good1/Kalman estimator cos 1 sin 0 ==
  flux : Inport
  ialp : Inport  Port=2
  ibet : Inport  Port=3
  Valp : Inport  Port=4
  Vbet : Inport  Port=5
  the : Inport  Port=6
  xpr : Inport  Port=7
  Pkp : Inport  Port=8
  T : Inport  Port=9
  Clock : Clock
  Gain3 : Gain  Gain=2/P
  Kalman Equations : MATLAB Function  TreatAsAtomicUnit=on
  west : Outport
  thest : Outport  Port=2
  wmecest : Outport  Port=3
  ialpe : Outport  Port=4
  ibete : Outport  Port=5
  xprt : Outport  Port=6
  Pkpt : Outport  Port=7
  Out1 : Outport  Port=8
  Out2 : Outport  Port=9
  wires:
  Kalman Equations/7(K) -> Out2/1
  Kalman Equations/8(det0) -> Out1/1
  flux/1 -> Kalman Equations/1(f)
  Valp/1 -> Kalman Equations/4(valp)
  Vbet/1 -> Kalman Equations/5(vbet)
  Clock/1 -> Kalman Equations/7(tim)
  Kalman Equations/3(wrest) -> west/1, Gain3/1
  Kalman Equations/4(theest) -> thest/1
  Gain3/1 -> wmecest/1
  ialp/1 -> Kalman Equations/2(ialp)
  ibet/1 -> Kalman Equations/3(ibet)
  Kalman Equations/5(ialpest) -> ialpe/1
  Kalman Equations/6(ibetest) -> ibete/1
  Kalman Equations/1(xprt) -> xprt/1
  Kalman Equations/2(Pkpt) -> Pkpt/1
  the/1 -> Kalman Equations/6(the)
  xpr/1 -> Kalman Equations/8(xpr)
  Pkp/1 -> Kalman Equations/9(Pkp)
  T/1 -> Kalman Equations/11(T)

== system PMSM_z_domain_HDL/EKF/EKF good1/dq to alpha beta ==
  theta_r : Inport
  id : Inport  Port=2
  iq : Inport  Port=3
  Fcn : Fcn  Expr=cos(u(1))*u(2)-sin(u(1))*u(3)
  Fcn1 : Fcn  Expr=sin(u(1))*u(2)+cos(u(1))*u(3)
  Mux : Mux  Inputs=3
  ialpha : Outport
  ibeta : Outport  Port=2
  wires:
  Fcn/1 -> ialpha/1
  id/1 -> Mux/2
  Fcn1/1 -> ibeta/1
  theta_r/1 -> Mux/1
  iq/1 -> Mux/3
  Mux/1 -> Fcn1/1, Fcn/1

== matlab function PMSM_z_domain_HDL/EKF/EKF good1/Kalman estimator/Kalman Equations ==
  data: f input; xprt output; ialp input; ibet input; valp input; vbet input; thee input; tim input; Pkpt output; xpr input; Pkp input; wrest output; theest output; ialpest output; ibetest output; nois input; sampleTime input; K output; det0 output
function [xprt,Pkpt,wrest,theest,ialpest,ibetest,K,det0]     = fcn(f,ialp,ibet,valp,vbet,thee,tim,xpr,Pkp,nois,sampleTime)
%#eml

% xprt=[0;0;0;0];
%     Pkpt=[0.1 0 0 0;0 0.1 0 0;0 0 0.1 0;0 0 0 0.1];
if tim==0
    xprt=[0.1;0.1;0.1;0.1];
    tim;
    Pkpt=[5 0 0 0;0 5 0 0;0 0 10 0;0 0 0 1];
    wrest=0;
    theest=0;
    thee=0;
    ialpest=0;
    ibetest=0;
    wef=0;
    K=[0 0; 0 0; 0 0; 0 0];
    det0 = 0;
    thrq=0;
end

%Q=.085,.085, 15.2,0 gives same as .01,.01,5.2,0 same as .2,.2.45.2,0
Q=[0.01 0 0 0;0 .01 0 0;0 0 10 0;0 0 0 .001];


J = 0.0027;
B = 0.0136;
r=1.477;
Ld=19.75e-3;
p=8;
Lq=22.5e-3;
Ts=sampleTime;
L1=(Ld+Lq)/2;
L2=(Ld-Lq)/2;

%Tef=(3*p/4)*(f*iqest+(Ld-Lq)*idest*iqest);
ial=xpr(1,1);
ibe=xpr(2,1);
we=xpr(3,1);
thee=xpr(4,1);


I=[1 0 0 0;0 1 0 0;0 0 1 0;0 0 0 1];

xe=[ial+((valp/L1)-(r*ial/L1)+(we*f*sin(thee)/L1))*Ts;
    ibe+((vbet/L1)-(r*ibe/L1)-(we*f*cos(thee)/L1))*Ts;
    we;
    thee+(we*Ts)];

F=[1-(r*Ts/L1) 0 (Ts*f*sin(thee))/L1 (we*f*cos(thee)*Ts)/L1;
    0 1-(r*Ts/L1) -(Ts*f*cos(thee))/L1 (we*f*sin(thee)*Ts)/L1;
    0 0 1 0;
    0 0 Ts 1];%
% G=[1-(Ts/taud) Ts*xpr(3,1)*Lq/Ld Ts*Lq*xe(2,1)/Ld 0;
%     -Ld*Ts*xpr(3,1)/Lq 1-(Ts/tauq) Ts*(((-Ld/Lq)*xe(1,1))-(f/Lq)) 0;
%     (3*p/4)*((Ld-Lq)*xpr(2,1))*Ts (3*p/4)*(f+(Ld-Lq)*xpr(1,1))*Ts 1-((B/J)*Ts) 0;
%     0 0 Ts 1];

% end
Rd=0.92;
R=[Rd 0;0 Rd];
%noise=sqrt(Rd/7)*randn;
yk=[ialp;ibet];%+[noise;noise];
C=[1 0 0 0;
    0 1 0 0];
Pk=F*Pkp*transpose(F)+Q;
K=Pk*transpose(C)/(C*Pk*transpose(C)+R);
x=xe+K*(yk-C*xe);
P=(I-K*C)*Pk;
det0 = det(C*Pk*transpose(C)+R);
xprt=I*x;
Pkpt=I*P;
wrest=x(3,1);
theest=x(4,1);
ialpest=x(1,1);
ibetest=x(2,1);
end

== matlab function PMSM_z_domain_HDL/EKF/EKF good/MATLAB Function ==
  data: u input; ymk input; Lambda_m input; Ls input; Rs input; x_prev input; P_prev input; P output; x output; t input; T input
function [P,x] = fcn(u, ymk,Lambda_m,Ls,Rs,x_prev,P_prev,t,T)


Ts=T;

B = [1/Ls 0;
    0 1/Ls;
    0 0;
    0 0];

Q = [0.1 0 0 0;
    0 0.1 0 0;
    0 0 25 0;
    0 0 0 0.0001];
R = [0.01 0;
    0 0.01];

P0=[5 0 0 0;
    0 5 0 0;
    0 0 100 0;
    0 0 0 1];
H = [1 0 0 0;
    0 1 0 0];


if t == 0
    P = P0;
    x = [0;
        0;
        0;
        0];


else
    
i_alpha = x_prev(1);
i_beta = x_prev(2);
omega = x_prev(3);
theta = x_prev(4);

Fx=[-Rs*i_alpha/Ls + (omega*Lambda_m/Ls)*sin(theta);
    -Rs*i_beta/Ls - (omega*Lambda_m/Ls)*cos(theta);
    0;
    omega];
    
%Compute jacobian matrix

Fk = [-Rs/Ls 0 Lambda_m*sin(theta)/Ls Lambda_m*omega*cos(theta)/Ls;
        0 -Rs/Ls -Lambda_m*cos(theta)/Ls Lambda_m*omega*sin(theta)/Ls;
        0 0 0 0;
        0 0 1 0];


% 1 )Update new mean
x_e = x_prev + Fx*Ts +B*u*Ts;

% 2) Estimation error covariance :

P_e = P_prev + (Fk*P_prev + P_prev*transpose(Fk))*Ts + Q;

%3) Predicted output :
ypk = H*x_e;

%4) Calculate kalman gain

K = P_e*transpose(H)/((H*P_e*transpose(H) + R));

%5) update state and error covariances

x_e = x_e + K*(ymk-ypk);
P_e = (eye(4)-K*H)*P_e*transpose(eye(4)-K*H)+K*R*transpose(K);
P = P_e;
x = x_e;
y_predicted=ypk;
end

== matlab function PMSM_z_domain_HDL/EKF/EKF good1/MATLAB Function ==
  data: u input; ymk input; Lambda_m input; Ls input; Rs input; x_prev input; P_prev input; P output; x output; t input; T input
function [P,x] = fcn(u, ymk,Lambda_m,Ls,Rs,x_prev,P_prev,t,T)


Ts=T;

B = [1/Ls 0;
    0 1/Ls;
    0 0;
    0 0];

Q = [0.1 0 0 0;
    0 0.1 0 0;
    0 0 25 0;
    0 0 0 0.0001];
R = [0.01 0;
    0 0.01];

P0=[5 0 0 0;
    0 5 0 0;
    0 0 5 0;
    0 0 0 1];
H = [1 0 0 0;
    0 1 0 0];


if t == 0
    P = P0;
    x = [0;
        0;
        0;
        0];


else
    
i_alpha = x_prev(1);
i_beta = x_prev(2);
omega = x_prev(3);
theta = x_prev(4);

Fx=[-Rs*i_alpha/Ls + (omega*Lambda_m/Ls)*sin(theta);
    -Rs*i_beta/Ls - (omega*Lambda_m/Ls)*cos(theta);
    0;
    omega];
    
%Compute jacobian matrix

Fk = [-Rs/Ls 0 Lambda_m*sin(theta)/Ls Lambda_m*omega*cos(theta)/Ls;
        0 -Rs/Ls -Lambda_m*cos(theta)/Ls Lambda_m*omega*sin(theta)/Ls;
        0 0 0 0;
        0 0 1 0];


% 1 )Update new mean
x_e = x_prev + Fx*Ts +B*u*Ts;

% 2) Estimation error covariance :

P_e = P_prev + (Fk*P_prev + P_prev*transpose(Fk))*Ts + Q;

%3) Predicted output :
ypk = H*x_e;

%4) Calculate kalman gain

K = P_e*transpose(H)/((H*P_e*transpose(H) + R));

%5) update state and error covariances

x_e = x_e + K*(ymk-ypk);
P_e = (eye(4)-K*H)*P_e*transpose(eye(4)-K*H)+K*R*transpose(K);
P = P_e;
x = x_e;
y_predicted=ypk;
end

== matlab function PMSM_z_domain_HDL/EKF/EKF good1/Kalman estimator cos 1 sin 0/Kalman Equations ==
  data: f input; xprt output; ialp input; ibet input; valp input; vbet input; the input; tim input; Pkpt output; xpr input; Pkp input; wrest output; theest output; ialpest output; ibetest output; nois input; T input; K output; det0 output
function [xprt,Pkpt,wrest,theest,ialpest,ibetest,K,det0]     = fcn(f,ialp,ibet,valp,vbet,the,tim,xpr,Pkp,nois,T)
%#eml
I=[1 0 0 0;0 1 0 0;0 0 1 0;0 0 0 1];

% xprt=[0;0;0;0];
%     Pkpt=[0.1 0 0 0;0 0.1 0 0;0 0 0.1 0;0 0 0 0.1];
if tim==0
    xprt=[1;1;0;0];
    tim;
    Pkpt=[5 0 0 0;0 5 0 0;0 0 100 0;0 0 0 1];
    wrest=0;
    theest=0;
    ialpest=0;
    ibetest=0;
    wef=0;
    K=[0 0; 0 0; 0 0; 0 0];
    det0 = 0;
    thrq=0;
end
if tim<.1
    Qs=1;
else
    Qs=1;
end
%Q=.085,.085, 15.2,0 gives same as .01,.01,5.2,0 same as .2,.2.45.2,0
Q=[.01 0 0 0;0 .01 0 0;0 0 Qs 0;0 0 0 .0001];


J=1.58061e-3;
B=3.4e-3;
r=1.477;
Ld=19.75e-3;
p=8;
Lq=22.5e-3;
Ts=T;
L1=(Ld+Lq)/2;
L2=(Ld-Lq)/2;

%Tef=(3*p/4)*(f*iqest+(Ld-Lq)*idest*iqest);
ial=xpr(1,1);
ibe=xpr(2,1);
we=xpr(3,1);
if tim<1e-4
    thee=0;
else
thee=xpr(4,1);
end
% Tef=f*((-ial*sin(thee)+ibe*cos(thee)))+((Ld-Lq)*(ial*cos(thee)+ibe*sin(thee))*(-ial*sin(thee)+ibe*cos(thee)));

I=[1 0 0 0;0 1 0 0;0 0 1 0;0 0 0 1];

xe=[ial+((valp/L1)-(r*ial/L1)+(we*f*sin(0)/L1))*Ts;
    ibe+((vbet/L1)-(r*ibe/L1)-(we*f*cos(0)/L1))*Ts;
    we;
    thee+(we*Ts)];

F=[1-(r*Ts/L1) 0 (Ts*f*sin(thee))/L1 (we*f*cos(0)*Ts)/L1;
    0 1-(r*Ts/L1) -(Ts*f*cos(thee))/L1 (we*f*sin(0)*Ts)/L1;
    0 0 1 0;
    0 0 Ts 1];%
% G=[1-(Ts/taud) Ts*xpr(3,1)*Lq/Ld Ts*Lq*xe(2,1)/Ld 0;
%     -Ld*Ts*xpr(3,1)/Lq 1-(Ts/tauq) Ts*(((-Ld/Lq)*xe(1,1))-(f/Lq)) 0;
%     (3*p/4)*((Ld-Lq)*xpr(2,1))*Ts (3*p/4)*(f+(Ld-Lq)*xpr(1,1))*Ts 1-((B/J)*Ts) 0;
%     0 0 Ts 1];

% end
Rd=0.92;
R=[Rd 0;0 Rd];
%noise=sqrt(Rd/7)*randn;
yk=[ialp;ibet];%+[noise;noise];
C=[1 0 0 0;
    0 1 0 0];
Pk=F*Pkp*transpose(F)+Q;
K=Pk*transpose(C)/(C*Pk*transpose(C)+R);
x=xe+K*(yk-C*xe);
P=(I-K*C)*Pk;
det0 = det(C*Pk*transpose(C)+R);
xprt=I*x;
Pkpt=I*P;
wrest=x(3,1);
theest=x(4,1);
ialpest=x(1,1);
ibetest=x(2,1);
end

== matlab function PMSM_z_domain_HDL/EKF/EKF good/Kalman estimator/Kalman Equations ==
  data: f input; xprt output; ialp input; ibet input; valp input; vbet input; the input; tim input; Pkpt output; xpr input; Pkp input; wrest output; theest output; ialpest output; ibetest output; nois input; T input
function [xprt,Pkpt,wrest,theest,ialpest,ibetest]     = fcn(f,ialp,ibet,valp,vbet,the,tim,xpr,Pkp,nois,T)
%#eml
I=[1 0 0 0;0 1 0 0;0 0 1 0;0 0 0 1];

% xprt=[0;0;0;0];
%     Pkpt=[0.1 0 0 0;0 0.1 0 0;0 0 0.1 0;0 0 0 0.1];
if tim==0
    xprt=[1;1;0;0];
    tim;
    Pkpt=[5 0 0 0;0 5 0 0;0 0 100 0;0 0 0 1];
    wrest=0;
    theest=0;
    ialpest=0;
    ibetest=0;
    wef=0;
    
    thrq=0;
end
if tim<.1
    Qs=20;
else
    Qs=20;
end
%Q=.085,.085, 15.2,0 gives same as .01,.01,5.2,0 same as .2,.2.45.2,0
Q=[.01 0 0 0;0 .01 0 0;0 0 Qs 0;0 0 0 .0001];


J=1.58061e-3;
B=3.4e-3;
r=1.477;
Ld=19.75e-3;
p=8;
Lq=22.5e-3;
Ts=T;
L1=(Ld+Lq)/2;
L2=(Ld-Lq)/2;

%Tef=(3*p/4)*(f*iqest+(Ld-Lq)*idest*iqest);
ial=xpr(1,1);
ibe=xpr(2,1);
we=xpr(3,1);
if tim<1e-4
    thee=0;
else
thee=xpr(4,1);
end
% Tef=f*((-ial*sin(thee)+ibe*cos(thee)))+((Ld-Lq)*(ial*cos(thee)+ibe*sin(thee))*(-ial*sin(thee)+ibe*cos(thee)));

I=[1 0 0 0;0 1 0 0;0 0 1 0;0 0 0 1];

xe=[ial+((valp/L1)-(r*ial/L1)+(we*f*sin(thee)/L1))*Ts;
    ibe+((vbet/L1)-(r*ibe/L1)-(we*f*cos(thee)/L1))*Ts;
    we;
    thee+(we*Ts)];

F=[1-(r*Ts/L1) 0 (Ts*f*sin(thee))/L1 (we*f*cos(thee)*Ts)/L1;
    0 1-(r*Ts/L1) -(Ts*f*cos(thee))/L1 (we*f*sin(thee)*Ts)/L1;
    0 0 1 0;
    0 0 Ts 1];%
% G=[1-(Ts/taud) Ts*xpr(3,1)*Lq/Ld Ts*Lq*xe(2,1)/Ld 0;
%     -Ld*Ts*xpr(3,1)/Lq 1-(Ts/tauq) Ts*(((-Ld/Lq)*xe(1,1))-(f/Lq)) 0;
%     (3*p/4)*((Ld-Lq)*xpr(2,1))*Ts (3*p/4)*(f+(Ld-Lq)*xpr(1,1))*Ts 1-((B/J)*Ts) 0;
%     0 0 Ts 1];

% end
Rd=1;
R=[Rd 0;0 Rd];
%noise=sqrt(Rd/7)*randn;
yk=[ialp;ibet];%+[noise;noise];
C=[1 0 0 0;
    0 1 0 0];
Pk=F*Pkp*transpose(F)+Q;
K=Pk*transpose(C)/(C*Pk*transpose(C)+R);
x=xe+K*(yk-C*xe);
P=(I-K*C)*Pk;
xprt=I*x;
Pkpt=I*P;
wrest=x(3,1);
theest=x(4,1);
ialpest=x(1,1);
ibetest=x(2,1);
end
